simulink model "controlador_multirate"  (R2012b)
settings: Solver=ode3  StartTime=0.0  StopTime=1  FixedStep=1e-5  RelTol=1e-3
model workspace: external: MATLAB File Z:\Work\PLATO\2 - simulador BLDC\3 - Simulador controlador multirate\5 - compacao multirate, sensor MT x sensor M x sensor T\config_simulador_BLDC.m (data not in the file)
undefined symbols (not defined in the file): J, Kd, Ke, Kt, L, Nr, P, R
libraries: simulink x71
(part 1 of 2)
settings Model: Creator=Juliano  LastModifiedBy=Juliano

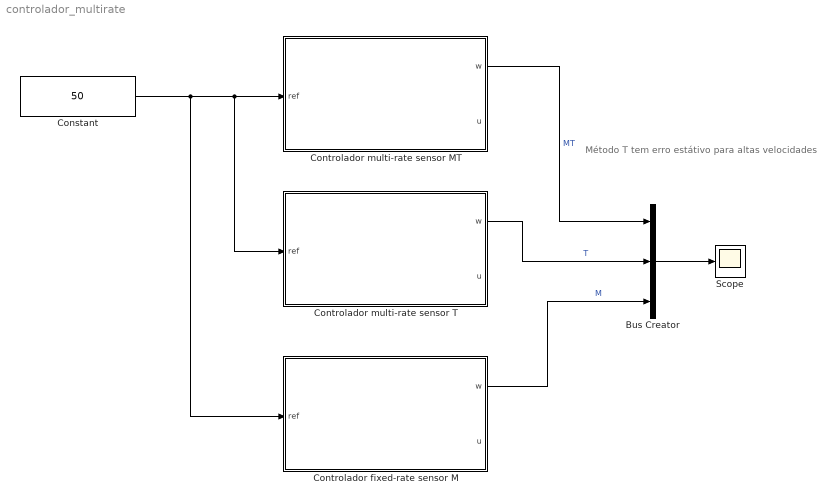
== system controlador_multirate ==
  note: Método T tem erro estátivo para altas velocidades
  Bus Creator : BusCreator  Inputs=3
  Constant : Constant  Value=50
  Controlador fixed-rate sensor M : Subsystem  mask{Ts=0.01}
      mask prompts: Ts "Sample Time"
  Controlador multi-rate sensor MT : Subsystem  mask{Ts=0.01}
      mask prompts: Ts "Sample time inicial do método M/T"
  Controlador multi-rate sensor T : Subsystem  mask{m=10}
      mask prompts: m "Número de pulsos que o método T espera para dar uma estimativa de velocidade (m)"
  Scope : Scope
      settings: TickLabels=on  ShowLegends=on  YMin=5  YMax=85
  wires:
  Constant/1 -> Controlador fixed-rate sensor M/1(ref), Controlador multi-rate sensor T/1(ref), Controlador multi-rate sensor MT/1(ref)
  Controlador multi-rate sensor MT/1(w) -> Bus Creator/1  "MT"
  Controlador fixed-rate sensor M/1(w) -> Bus Creator/3  "M"
  Bus Creator/1 -> Scope/1
  Controlador multi-rate sensor T/1(w) -> Bus Creator/2  "T"

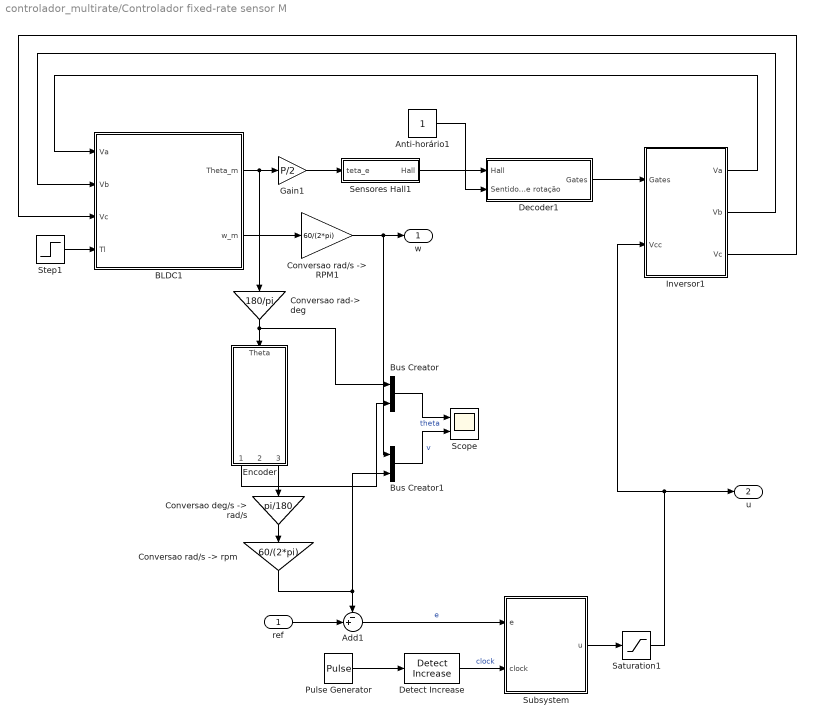
== system controlador_multirate/Controlador fixed-rate sensor M ==
  ref : Inport
  Add1 : Sum  Inputs=-+|
  Anti-horário1 : Constant
  BLDC1 : Subsystem
  Bus Creator : BusCreator  Inputs=2
  Bus Creator1 : BusCreator  Inputs=2
  "Conversao deg/s -> rad/s" : Gain  Gain=pi/180
  Conversao rad-> deg : Gain  Gain=180/pi
  "Conversao rad/s -> RPM1" : Gain  Gain=60/(2*pi)
  "Conversao rad/s -> rpm" : Gain  Gain=60/(2*pi)
  Decoder1 : Subsystem
  Detect Increase : simulink/Logic and Bit Operations/Detect Increase  vinit=0.0  InputProcessing=Inherited  OutDataTypeStr=boolean
  Encoder : Subsystem  mask{Nr=Nr}
      mask prompts: Nr "Número de pulsos por revolução"
  Gain1 : Gain  Gain=P/2
  Inversor1 : Subsystem
  Pulse Generator : DiscretePulseGenerator  PulseType=Time based  Period=Ts  PulseWidth=50
  Saturation1 : Saturate  UpperLimit=12  LowerLimit=-12
  Scope : Scope  NumInputPorts=2
      settings: ShowLegends=on  YMin=0~-350  YMax=400~600
  Sensores Hall1 : Subsystem  AncestorBlock=spsPMSynchronousMachineModel/Discrete Trapezoidal/Hall effect sensor
  Step1 : Step  Time=0.2  After=0*2e-3  SampleTime=0
  Subsystem : Subsystem
  w : Outport
  u : Outport  Port=2
  wires:
  BLDC1/2(w_m) -> "Conversao rad/s -> RPM1"/1
  Inversor1/3(Vc) -> BLDC1/3(Vc)
  Subsystem/1(u) -> Saturation1/1
  Gain1/1 -> Sensores Hall1/1(teta_e)
  "Conversao deg/s -> rad/s"/1 -> "Conversao rad/s -> rpm"/1
  Add1/1 -> Subsystem/1(e)  "e"
  BLDC1/1(Theta_m) -> Gain1/1, Conversao rad-> deg/1
  Step1/1 -> BLDC1/4(Tl)
  Sensores Hall1/1(Hall) -> Decoder1/1("Hall ")
  Inversor1/2(Vb) -> BLDC1/2(Vb)
  Inversor1/1(Va) -> BLDC1/1(Va)
  Decoder1/1(Gates) -> Inversor1/1(Gates)
  Anti-horário1/1 -> Decoder1/2(Sentido de rotação)
  Detect Increase/1 -> Subsystem/2(clock)  "clock"
  Saturation1/1 -> u/1, Inversor1/2(Vcc)
  ref/1 -> Add1/2
  Encoder/3(VelocidadeM) -> "Conversao deg/s -> rad/s"/1
  Pulse Generator/1 -> Detect Increase/1
  Conversao rad-> deg/1 -> Bus Creator/1, Encoder/1(Theta)
  "Conversao rad/s -> rpm"/1 -> Add1/1, Bus Creator1/2
  "Conversao rad/s -> RPM1"/1 -> Bus Creator1/1, w/1
  Encoder/1(Theta_amostrado) -> Bus Creator/2
  Bus Creator/1 -> Scope/1  "theta"
  Bus Creator1/1 -> Scope/2  "v"

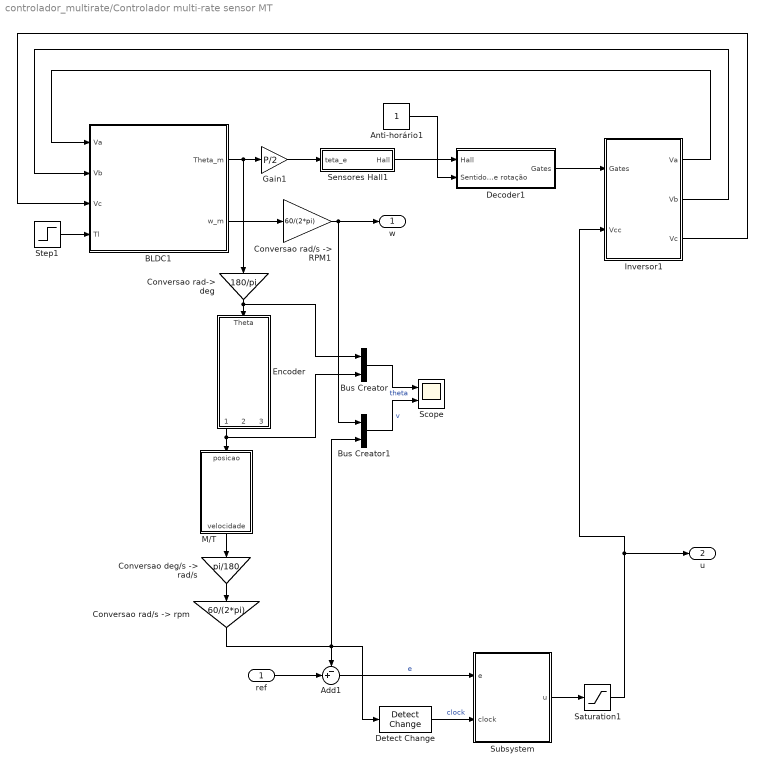
== system controlador_multirate/Controlador multi-rate sensor MT ==
  ref : Inport
  Add1 : Sum  Inputs=-+|
  Anti-horário1 : Constant
  BLDC1 : Subsystem
  Bus Creator : BusCreator  Inputs=2
  Bus Creator1 : BusCreator  Inputs=2
  "Conversao deg/s -> rad/s" : Gain  Gain=pi/180
  Conversao rad-> deg : Gain  Gain=180/pi
  "Conversao rad/s -> RPM1" : Gain  Gain=60/(2*pi)
  "Conversao rad/s -> rpm" : Gain  Gain=60/(2*pi)
  Decoder1 : Subsystem
  Detect Change : simulink/Logic and Bit Operations/Detect Change  vinit=1  InputProcessing=Inherited  OutDataTypeStr=boolean
  Encoder : Subsystem  mask{Nr=Nr}
      mask prompts: Nr "Número de pulsos por revolução"
  Gain1 : Gain  Gain=P/2
  Inversor1 : Subsystem
  M/T : Subsystem  mask{Ts=Ts}
      mask prompts: Ts "Sampling time"
  Saturation1 : Saturate  UpperLimit=12  LowerLimit=-12
  Scope : Scope  NumInputPorts=2
      settings: ShowLegends=on  YMin=0~-350  YMax=400~600  SaveName=ScopeData8
  Sensores Hall1 : Subsystem  AncestorBlock=spsPMSynchronousMachineModel/Discrete Trapezoidal/Hall effect sensor
  Step1 : Step  Time=0.2  After=0*2e-3  SampleTime=0
  Subsystem : Subsystem
  w : Outport
  u : Outport  Port=2
  wires:
  BLDC1/2(w_m) -> "Conversao rad/s -> RPM1"/1
  Inversor1/3(Vc) -> BLDC1/3(Vc)
  Subsystem/1(u) -> Saturation1/1
  Gain1/1 -> Sensores Hall1/1(teta_e)
  "Conversao deg/s -> rad/s"/1 -> "Conversao rad/s -> rpm"/1
  Add1/1 -> Subsystem/1(e)  "e"
  Conversao rad-> deg/1 -> Bus Creator/1, Encoder/1(Theta)
  BLDC1/1(Theta_m) -> Gain1/1, Conversao rad-> deg/1
  Step1/1 -> BLDC1/4(Tl)
  "Conversao rad/s -> rpm"/1 -> Bus Creator1/2, Add1/1, Detect Change/1
  Sensores Hall1/1(Hall) -> Decoder1/1("Hall ")
  Inversor1/2(Vb) -> BLDC1/2(Vb)
  Inversor1/1(Va) -> BLDC1/1(Va)
  Decoder1/1(Gates) -> Inversor1/1(Gates)
  Anti-horário1/1 -> Decoder1/2(Sentido de rotação)
  Detect Change/1 -> Subsystem/2(clock)  "clock"
  Saturation1/1 -> u/1, Inversor1/2(Vcc)
  ref/1 -> Add1/2
  "Conversao rad/s -> RPM1"/1 -> w/1, Bus Creator1/1
  Encoder/1(Theta_amostrado) -> Bus Creator/2, M/T/1(posicao)
  M/T/1(velocidade) -> "Conversao deg/s -> rad/s"/1
  Bus Creator/1 -> Scope/1  "theta"
  Bus Creator1/1 -> Scope/2  "v"

== system controlador_multirate/Controlador multi-rate sensor T ==
  ref : Inport
  Add1 : Sum  Inputs=-+|
  Anti-horário1 : Constant
  BLDC1 : Subsystem
  Bus Creator : BusCreator  Inputs=2
  Bus Creator1 : BusCreator  Inputs=2
  "Conversao deg/s -> rad/s" : Gain  Gain=pi/180
  Conversao rad-> deg : Gain  Gain=180/pi
  "Conversao rad/s -> RPM1" : Gain  Gain=60/(2*pi)
  "Conversao rad/s -> rpm" : Gain  Gain=60/(2*pi)
  Decoder1 : Subsystem
  Detect Change : simulink/Logic and Bit Operations/Detect Change  vinit=1  InputProcessing=Inherited  OutDataTypeStr=boolean
  Encoder : Subsystem  mask{Nr=Nr}
      mask prompts: Nr "Número de pulsos por revolução"
  Gain1 : Gain  Gain=P/2
  Inversor1 : Subsystem
  Saturation1 : Saturate  UpperLimit=12  LowerLimit=-12
  Scope : Scope  NumInputPorts=2
      settings: ShowLegends=on  YMin=0~-400  YMax=275~450  SaveName=ScopeData7
  Sensores Hall1 : Subsystem  AncestorBlock=spsPMSynchronousMachineModel/Discrete Trapezoidal/Hall effect sensor
  Step1 : Step  Time=0.2  After=0*2e-3  SampleTime=0
  Subsystem : Subsystem
  w : Outport
  u : Outport  Port=2
  wires:
  BLDC1/2(w_m) -> "Conversao rad/s -> RPM1"/1
  Inversor1/3(Vc) -> BLDC1/3(Vc)
  Subsystem/1(u) -> Saturation1/1
  Gain1/1 -> Sensores Hall1/1(teta_e)
  "Conversao deg/s -> rad/s"/1 -> "Conversao rad/s -> rpm"/1
  Add1/1 -> Subsystem/1(e)  "e"
  BLDC1/1(Theta_m) -> Gain1/1, Conversao rad-> deg/1
  Step1/1 -> BLDC1/4(Tl)
  "Conversao rad/s -> rpm"/1 -> Bus Creator1/2, Add1/1, Detect Change/1
  Sensores Hall1/1(Hall) -> Decoder1/1("Hall ")
  Inversor1/2(Vb) -> BLDC1/2(Vb)
  Inversor1/1(Va) -> BLDC1/1(Va)
  Decoder1/1(Gates) -> Inversor1/1(Gates)
  Anti-horário1/1 -> Decoder1/2(Sentido de rotação)
  Detect Change/1 -> Subsystem/2(clock)  "clock"
  Saturation1/1 -> u/1, Inversor1/2(Vcc)
  ref/1 -> Add1/2
  Encoder/2(VelocidadeT) -> "Conversao deg/s -> rad/s"/1
  Conversao rad-> deg/1 -> Bus Creator/1, Encoder/1(Theta)
  "Conversao rad/s -> RPM1"/1 -> Bus Creator1/1, w/1
  Encoder/1(Theta_amostrado) -> Bus Creator/2
  Bus Creator/1 -> Scope/1  "theta"
  Bus Creator1/1 -> Scope/2  "v"

== system controlador_multirate/Controlador fixed-rate sensor M/BLDC1 ==
  Va : Inport
  Vb : Inport  Port=2
  Vc : Inport  Port=3
  Tl : Inport  Port=4
  "Cálculo Torque fase \"a\"" : Subsystem
  "Cálculo Torque fase \"b\"" : Subsystem
  "Cálculo Torque fase \"c\"" : Subsystem
  Cálculo das FCEMs : Subsystem
  "Dinâmica fase \"a\"" : Subsystem
  "Dinâmica fase \"b\"" : Subsystem
  "Dinâmica fase \"c\"" : Subsystem
  "Dinâmica mecânica " : Subsystem
  FCEMs : Scope  NumInputPorts=3
      settings: TimeRange=1  YMin=420~-5~-5  YMax=510~5~5  SaveName=ScopeData5
  Gain2 : Gain  Gain=P/2
  Scope : Scope
      settings: TimeRange=1  YMin=420  YMax=510  SaveName=ScopeData4
  Sum : Sum  Inputs=+++
  Vs : Scope  NumInputPorts=3
      settings: TimeRange=1  YMin=420~-5~-5  YMax=510~5~5  SaveName=ScopeData2
  is : Scope  NumInputPorts=3
      settings: TimeRange=1  YMin=420~-5~-5  YMax=510~5~5  SaveName=ScopeData3
  is1 : Scope  NumInputPorts=3
      settings: TimeRange=1  YMin=420~-5~-5  YMax=510~5~5  SaveName=ScopeData6
  Theta_m : Outport
  w_m : Outport  Port=2
  wires:
  Gain2/1 -> "Cálculo Torque fase \"b\""/2(Theta_e), Cálculo das FCEMs/1(Theta_e), "Cálculo Torque fase \"c\""/2(Theta_e), "Cálculo Torque fase \"a\""/2(Theta_e)
  Tl/1 -> "Dinâmica mecânica "/2(Tl)
  "Dinâmica mecânica "/2(w_m) -> w_m/1, Cálculo das FCEMs/2(w_m)  "w_m"
  "Dinâmica mecânica "/1(Theta_m) -> Gain2/1, Theta_m/1  "Theta_m"
  Sum/1 -> "Dinâmica mecânica "/1(Te), Scope/1  "T"
  "Cálculo Torque fase \"c\""/1(T_c) -> Sum/3, is1/3  "T_c"
  "Cálculo Torque fase \"b\""/1(T_b) -> Sum/2, is1/2  "T_b"
  "Cálculo Torque fase \"a\""/1(T_a) -> Sum/1, is1/1  "T_a"
  "Dinâmica fase \"c\""/1(i_c) -> "Cálculo Torque fase \"c\""/1(i_c), is/3  "i_c"
  "Dinâmica fase \"b\""/1(i_b) -> "Cálculo Torque fase \"b\""/1(i_b), is/2  "i_b"
  "Dinâmica fase \"a\""/1(i_a) -> "Cálculo Torque fase \"a\""/1(i_a), is/1  "i_a"
  Vc/1 -> "Dinâmica fase \"c\""/1(Vc), Vs/3
  Vb/1 -> "Dinâmica fase \"b\""/1(Vb), Vs/2
  Va/1 -> "Dinâmica fase \"a\""/1(Va), Vs/1
  Cálculo das FCEMs/3(e_c) -> "Dinâmica fase \"c\""/2(e_c), FCEMs/3  "e_c"
  Cálculo das FCEMs/2(e_b) -> FCEMs/2, "Dinâmica fase \"b\""/2(e_b)  "e_b"
  Cálculo das FCEMs/1(e_a) -> "Dinâmica fase \"a\""/2(e_a), FCEMs/1  "e_a"

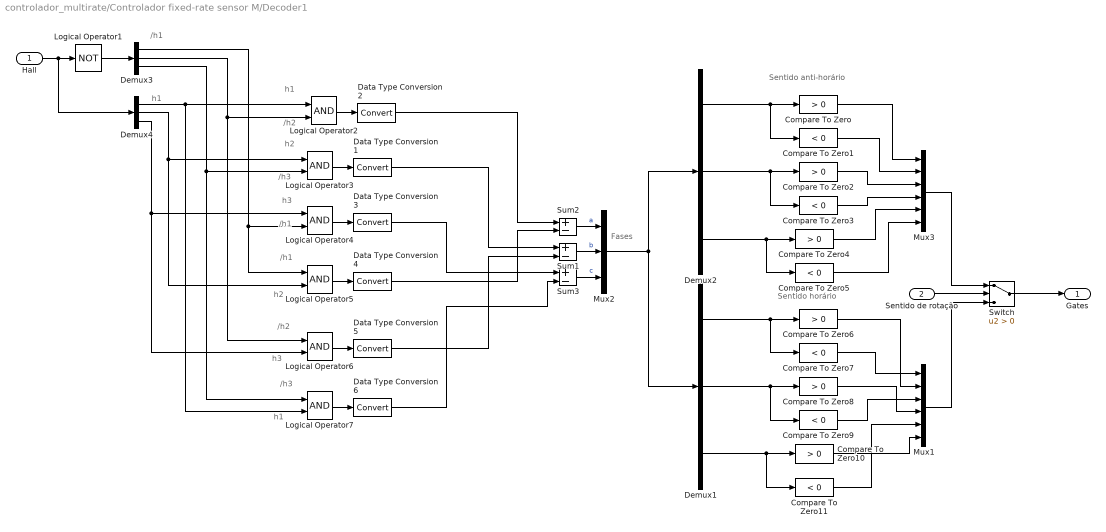
== system controlador_multirate/Controlador fixed-rate sensor M/Decoder1 ==
  note: /h1
  note: h1
  note: h1
  note: /h2
  note: h2
  note: /h3
  note: h3
  note: /h1
  note: /h1
  note: h2
  note: /h2
  note: h3
  note: /h3
  note: h1
  note: Sentido anti-horário
  note: Sentido horário
  note: Fases
  "Hall " : Inport
  Sentido de rotação : Inport  Port=2
  Compare To Zero{,2,4,6,8,10} (6 alike) : simulink/Logic and Bit Operations/Compare To Zero  relop=>  OutDataTypeStr=boolean  ZeroCross=off
  Compare To Zero{1,3,5,7,9,11} (6 alike) : simulink/Logic and Bit Operations/Compare To Zero  relop=<  OutDataTypeStr=boolean  ZeroCross=off
  Data Type Conversion{1..6} (6 alike) : DataTypeConversion
  Demux{1..4} (4 alike) : Demux  Outputs=3
  Logical Operator1 : Logic  Operator=NOT  AllPortsSameDT=off  OutDataTypeStr=boolean
  Logical Operator{2..7} (6 alike) : Logic  AllPortsSameDT=off  OutDataTypeStr=boolean
  Mux1 : Mux  Inputs=6
  Mux2 : Mux  Inputs=3
  Mux3 : Mux  Inputs=6
  Sum1 : Sum  Inputs=+-  OutDataTypeStr=double
  Sum2 : Sum  Inputs=+-  OutDataTypeStr=double
  Sum3 : Sum  Inputs=+-  OutDataTypeStr=double
  Switch : Switch  Criteria=u2 > Threshold
  Gates : Outport
  wires:
  Demux2/1 -> Compare To Zero/1, Compare To Zero1/1
  Demux2/2 -> Compare To Zero2/1, Compare To Zero3/1
  Demux2/3 -> Compare To Zero4/1, Compare To Zero5/1
  Compare To Zero/1 -> Mux3/1
  Compare To Zero1/1 -> Mux3/2
  Compare To Zero2/1 -> Mux3/3
  Compare To Zero3/1 -> Mux3/4
  Compare To Zero4/1 -> Mux3/5
  Compare To Zero5/1 -> Mux3/6
  Demux1/1 -> Compare To Zero6/1, Compare To Zero7/1
  Demux1/2 -> Compare To Zero8/1, Compare To Zero9/1
  Demux1/3 -> Compare To Zero10/1, Compare To Zero11/1
  Mux3/1 -> Switch/1
  Sentido de rotação/1 -> Switch/2
  Mux1/1 -> Switch/3
  Switch/1 -> Gates/1
  Compare To Zero7/1 -> Mux1/1
  Compare To Zero6/1 -> Mux1/2
  Compare To Zero9/1 -> Mux1/3
  Compare To Zero8/1 -> Mux1/4
  Compare To Zero11/1 -> Mux1/5
  Compare To Zero10/1 -> Mux1/6
  "Hall "/1 -> Logical Operator1/1, Demux4/1
  Logical Operator1/1 -> Demux3/1
  Demux4/3 -> Logical Operator4/1, Logical Operator6/2
  Demux4/2 -> Logical Operator3/1, Logical Operator5/2
  Demux4/1 -> Logical Operator2/1, Logical Operator7/2
  Demux3/3 -> Logical Operator3/2, Logical Operator7/1
  Demux3/2 -> Logical Operator2/2, Logical Operator6/1
  Demux3/1 -> Logical Operator4/2, Logical Operator5/1
  Logical Operator2/1 -> Data Type Conversion2/1
  Sum2/1 -> Mux2/1  "a"
  Sum1/1 -> Mux2/2  "b"
  Sum3/1 -> Mux2/3  "c"
  Logical Operator3/1 -> Data Type Conversion1/1
  Logical Operator4/1 -> Data Type Conversion3/1
  Logical Operator5/1 -> Data Type Conversion4/1
  Logical Operator6/1 -> Data Type Conversion5/1
  Logical Operator7/1 -> Data Type Conversion6/1
  Data Type Conversion2/1 -> Sum2/1
  Data Type Conversion4/1 -> Sum2/2
  Data Type Conversion1/1 -> Sum1/1
  Data Type Conversion5/1 -> Sum1/2
  Data Type Conversion3/1 -> Sum3/1
  Data Type Conversion6/1 -> Sum3/2
  Mux2/1 -> Demux2/1, Demux1/1

== system controlador_multirate/Controlador fixed-rate sensor M/Encoder ==
  note: ATENÇÃO: Para o correto funcionamento desse encoder o step size da simulação deve ser menor do que 360/(4*Nr*Vmax),
      | onde Vmax é o valor máximo da derivada do Theta atigindo durante a simulação
  Theta : Inport
  Clock : Clock
  Derivative : Derivative
  Determinar direçao : Subsystem
  Fcn : Fcn  Expr=360/(4*Nr*u)
  Graus / pulso1 : Gain  Gain=360/(4*Nr)  OutDataTypeStr=double
  Memory : Memory  X0=-100
  Método M : Subsystem  mask{Ts=Ts}
      mask prompts: Ts "Sampling time"
  Método T : Subsystem  mask{m=10}
      mask prompts: m "Número de pulsos que o bloco espera para calcular a velocidade média"
  Relational Operator : RelationalOperator  Operator=>  OutDataTypeStr=boolean
  Sensor Óptico : Subsystem
  Sensor Óptico1 : Subsystem
  Stop Simulation : Stop
  Subsystem : Subsystem
  Sum : Sum  Inputs=|+-
  Theta_amostrado : Outport
  VelocidadeT : Outport  Port=2
  VelocidadeM : Outport  Port=3
  wires:
  Método M/1(Velocidade) -> VelocidadeM/1
  Método T/1(Velocidade) -> VelocidadeT/1
  Graus / pulso1/1 -> Theta_amostrado/1, Método T/3(Posição), Método M/1(Posição)
  Subsystem/1(Out) -> Graus / pulso1/1
  Determinar direçao/2(NEG) -> Subsystem/2(NEG)
  Determinar direçao/1(POS) -> Subsystem/1(POS)
  Sensor Óptico1/1(Sinal_Pulso) -> Determinar direçao/2(B), Método T/2(B)  "B"
  Sensor Óptico/1(Sinal_Pulso) -> Método T/1(A), Determinar direçao/1(A)  "A"
  Theta/1 -> Sensor Óptico/1(Theta), Derivative/1, Sensor Óptico1/1(Theta)
  Derivative/1 -> Relational Operator/1
  Clock/1 -> Memory/1, Sum/1
  Memory/1 -> Sum/2
  Sum/1 -> Fcn/1
  Fcn/1 -> Relational Operator/2
  Relational Operator/1 -> Stop Simulation/1

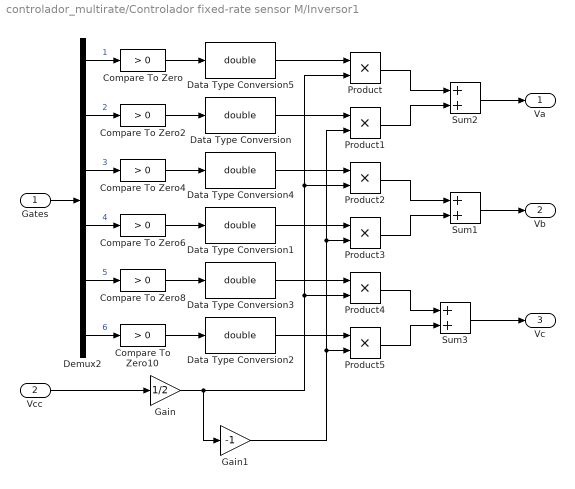
== system controlador_multirate/Controlador fixed-rate sensor M/Inversor1 ==
  Gates : Inport
  Vcc : Inport  Port=2
  Compare To Zero : simulink/Logic and Bit Operations/Compare To Zero  relop=>  OutDataTypeStr=uint8  ZeroCross=off
  Compare To Zero{2,6,8,10} (4 alike) : simulink/Logic and Bit Operations/Compare To Zero  relop=>  OutDataTypeStr=boolean  ZeroCross=off
  Compare To Zero4 : simulink/Logic and Bit Operations/Compare To Zero  relop=>  OutDataTypeStr=uint8  ZeroCross=off
  Data Type Conversion{,1..5} (6 alike) : DataTypeConversion  OutDataTypeStr=double
  Demux2 : Demux  Outputs=6
  Gain : Gain  Gain=1/2
  Gain1 : Gain  Gain=-1
  Product{,1..5} (6 alike) : Product  RndMeth=Zero
  Sum1 : Sum  SaturateOnIntegerOverflow=on
  Sum2 : Sum  SaturateOnIntegerOverflow=on
  Sum3 : Sum  SaturateOnIntegerOverflow=on
  Va : Outport
  Vb : Outport  Port=2
  Vc : Outport  Port=3
  wires:
  Gain/1 -> Product/2, Product2/2, Product4/2, Gain1/1
  Gain1/1 -> Product1/2, Product3/2, Product5/2
  Data Type Conversion5/1 -> Product/1
  Data Type Conversion/1 -> Product1/1
  Data Type Conversion4/1 -> Product2/1
  Data Type Conversion1/1 -> Product3/1
  Data Type Conversion3/1 -> Product4/1
  Data Type Conversion2/1 -> Product5/1
  Product5/1 -> Sum3/2
  Product4/1 -> Sum3/1
  Product3/1 -> Sum1/2
  Product2/1 -> Sum1/1
  Product1/1 -> Sum2/2
  Product/1 -> Sum2/1
  Compare To Zero10/1 -> Data Type Conversion2/1
  Compare To Zero8/1 -> Data Type Conversion3/1
  Compare To Zero6/1 -> Data Type Conversion1/1
  Compare To Zero4/1 -> Data Type Conversion4/1
  Compare To Zero2/1 -> Data Type Conversion/1
  Compare To Zero/1 -> Data Type Conversion5/1
  Demux2/6 -> Compare To Zero10/1  "6"
  Demux2/5 -> Compare To Zero8/1  "5"
  Demux2/4 -> Compare To Zero6/1  "4"
  Demux2/3 -> Compare To Zero4/1  "3"
  Demux2/2 -> Compare To Zero2/1  "2"
  Demux2/1 -> Compare To Zero/1  "1"
  Gates/1 -> Demux2/1
  Sum2/1 -> Va/1
  Sum3/1 -> Vc/1
  Sum1/1 -> Vb/1
  Vcc/1 -> Gain/1

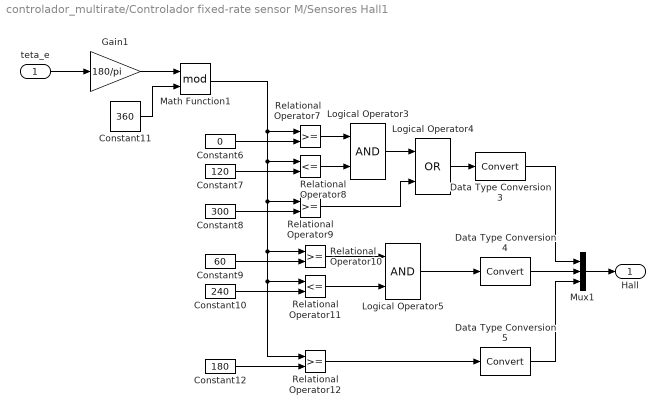
== system controlador_multirate/Controlador fixed-rate sensor M/Sensores Hall1 ==
  teta_e : Inport
  Constant10 : Constant  Value=240
  Constant11 : Constant  Value=360
  Constant12 : Constant  Value=180
  Constant6 : Constant  Value=0
  Constant7 : Constant  Value=120
  Constant8 : Constant  Value=300
  Constant9 : Constant  Value=60
  Data Type Conversion3 : DataTypeConversion  SaturateOnIntegerOverflow=on  RndMeth=Zero
  Data Type Conversion4 : DataTypeConversion  SaturateOnIntegerOverflow=on  RndMeth=Zero
  Data Type Conversion5 : DataTypeConversion  SaturateOnIntegerOverflow=on  RndMeth=Zero
  Gain1 : Gain  Gain=180/pi
  Logical Operator3 : Logic  AllPortsSameDT=off  OutDataTypeStr=boolean
  Logical Operator4 : Logic  Operator=OR  AllPortsSameDT=off  OutDataTypeStr=boolean
  Logical Operator5 : Logic  AllPortsSameDT=off  OutDataTypeStr=boolean
  Math Function1 : Math  Operator=mod  SaturateOnIntegerOverflow=on
  Mux1 : Mux  Inputs=3
  Relational Operator{7,9..10,12} (4 alike) : RelationalOperator  InputSameDT=on
  Relational Operator11 : RelationalOperator  Operator=<=  InputSameDT=on
  Relational Operator8 : RelationalOperator  Operator=<=  InputSameDT=on
  Hall : Outport
  wires:
  Math Function1/1 -> Relational Operator7/1, Relational Operator12/1, Relational Operator11/1, Relational Operator10/1, Relational Operator9/1, Relational Operator8/1
  Constant11/1 -> Math Function1/2
  Gain1/1 -> Math Function1/1
  Relational Operator12/1 -> Data Type Conversion5/1
  Logical Operator5/1 -> Data Type Conversion4/1
  Logical Operator4/1 -> Data Type Conversion3/1
  Data Type Conversion5/1 -> Mux1/3
  Data Type Conversion4/1 -> Mux1/2
  Data Type Conversion3/1 -> Mux1/1
  Mux1/1 -> Hall/1
  Constant12/1 -> Relational Operator12/2
  Constant10/1 -> Relational Operator11/2
  Constant9/1 -> Relational Operator10/2
  Relational Operator11/1 -> Logical Operator5/2
  Relational Operator10/1 -> Logical Operator5/1
  Relational Operator8/1 -> Logical Operator3/2
  Relational Operator7/1 -> Logical Operator3/1
  Logical Operator3/1 -> Logical Operator4/1
  Relational Operator9/1 -> Logical Operator4/2
  Constant8/1 -> Relational Operator9/2
  Constant7/1 -> Relational Operator8/2
  Constant6/1 -> Relational Operator7/2
  teta_e/1 -> Gain1/1

== system controlador_multirate/Controlador fixed-rate sensor M/Subsystem ==
  e : Inport
  clock : Inport  Port=2
  Clock : Clock
  Constant1 : Constant  Value=0.000518155
  Gain2 : Gain  Gain=0.0431726
  Gain3 : Gain  Gain=0.000518155
  Memória controlavel : Subsystem
  Memória controlavel (Y') : Subsystem
  Memória controlavel (e') : Subsystem
  Memória controlavel (u) : Subsystem
  Product : Product  RndMeth=Zero
  Sum : Sum  Inputs=++-
  Sum1 : Sum  Inputs=|+-
  Sum2 : Sum  Inputs=|+-
  u : Outport
  wires:
  e/1 -> Memória controlavel (e')/1(In), Gain3/1
  Memória controlavel (e')/1(Out) -> Product/1
  Memória controlavel (Y')/1(Out) -> Sum/1
  Gain2/1 -> Sum1/2
  clock/1 -> Memória controlavel (u)/2(ctrl), Memória controlavel/2(ctrl), Memória controlavel (e')/2(ctrl), Memória controlavel (Y')/2(ctrl)
  Sum/1 -> Memória controlavel (u)/1(In), Memória controlavel (Y')/1(In)
  Memória controlavel/1(Out) -> Sum2/2
  Product/1 -> Sum/3
  Gain3/1 -> Sum/2
  Clock/1 -> Sum2/1, Memória controlavel/1(In)
  Sum1/1 -> Product/2
  Constant1/1 -> Sum1/1
  Memória controlavel (u)/1(Out) -> u/1
  Sum2/1 -> Gain2/1

== system controlador_multirate/Controlador multi-rate sensor MT/BLDC1 ==
  Va : Inport
  Vb : Inport  Port=2
  Vc : Inport  Port=3
  Tl : Inport  Port=4
  "Cálculo Torque fase \"a\"" : Subsystem
  "Cálculo Torque fase \"b\"" : Subsystem
  "Cálculo Torque fase \"c\"" : Subsystem
  Cálculo das FCEMs : Subsystem
  "Dinâmica fase \"a\"" : Subsystem
  "Dinâmica fase \"b\"" : Subsystem
  "Dinâmica fase \"c\"" : Subsystem
  "Dinâmica mecânica " : Subsystem
  FCEMs : Scope  NumInputPorts=3
      settings: TimeRange=1  YMin=420~-5~-5  YMax=510~5~5  SaveName=ScopeData5
  Gain2 : Gain  Gain=P/2
  Scope : Scope
      settings: TimeRange=1  YMin=420  YMax=510  SaveName=ScopeData4
  Sum : Sum  Inputs=+++
  Vs : Scope  NumInputPorts=3
      settings: TimeRange=1  YMin=420~-5~-5  YMax=510~5~5  SaveName=ScopeData2
  is : Scope  NumInputPorts=3
      settings: TimeRange=1  YMin=420~-5~-5  YMax=510~5~5  SaveName=ScopeData3
  is1 : Scope  NumInputPorts=3
      settings: TimeRange=1  YMin=420~-5~-5  YMax=510~5~5  SaveName=ScopeData6
  Theta_m : Outport
  w_m : Outport  Port=2
  wires:
  Gain2/1 -> "Cálculo Torque fase \"b\""/2(Theta_e), Cálculo das FCEMs/1(Theta_e), "Cálculo Torque fase \"c\""/2(Theta_e), "Cálculo Torque fase \"a\""/2(Theta_e)
  Tl/1 -> "Dinâmica mecânica "/2(Tl)
  "Dinâmica mecânica "/2(w_m) -> w_m/1, Cálculo das FCEMs/2(w_m)  "w_m"
  "Dinâmica mecânica "/1(Theta_m) -> Gain2/1, Theta_m/1  "Theta_m"
  Sum/1 -> "Dinâmica mecânica "/1(Te), Scope/1  "T"
  "Cálculo Torque fase \"c\""/1(T_c) -> Sum/3, is1/3  "T_c"
  "Cálculo Torque fase \"b\""/1(T_b) -> Sum/2, is1/2  "T_b"
  "Cálculo Torque fase \"a\""/1(T_a) -> Sum/1, is1/1  "T_a"
  "Dinâmica fase \"c\""/1(i_c) -> "Cálculo Torque fase \"c\""/1(i_c), is/3  "i_c"
  "Dinâmica fase \"b\""/1(i_b) -> "Cálculo Torque fase \"b\""/1(i_b), is/2  "i_b"
  "Dinâmica fase \"a\""/1(i_a) -> "Cálculo Torque fase \"a\""/1(i_a), is/1  "i_a"
  Vc/1 -> "Dinâmica fase \"c\""/1(Vc), Vs/3
  Vb/1 -> "Dinâmica fase \"b\""/1(Vb), Vs/2
  Va/1 -> "Dinâmica fase \"a\""/1(Va), Vs/1
  Cálculo das FCEMs/3(e_c) -> "Dinâmica fase \"c\""/2(e_c), FCEMs/3  "e_c"
  Cálculo das FCEMs/2(e_b) -> FCEMs/2, "Dinâmica fase \"b\""/2(e_b)  "e_b"
  Cálculo das FCEMs/1(e_a) -> "Dinâmica fase \"a\""/2(e_a), FCEMs/1  "e_a"

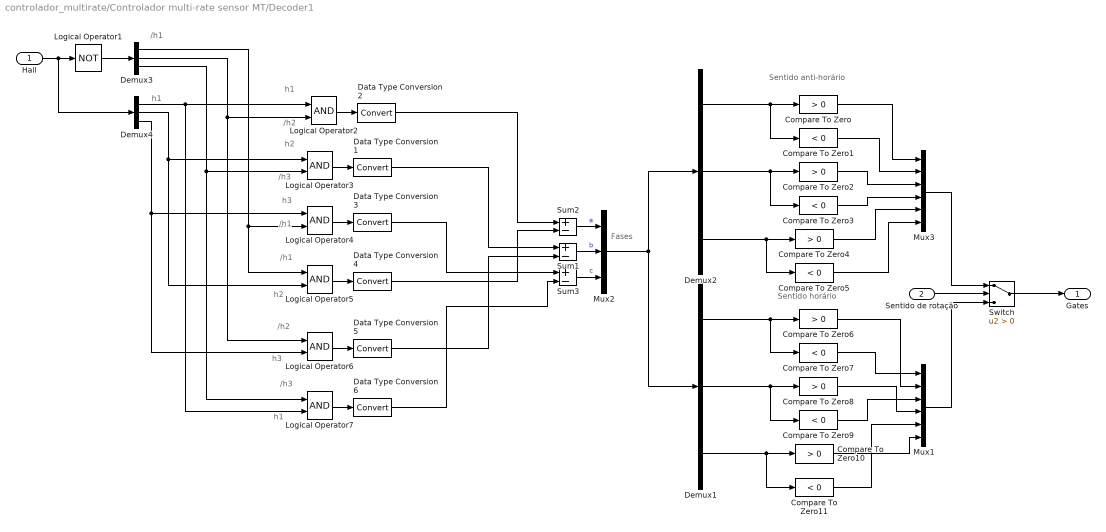
== system controlador_multirate/Controlador multi-rate sensor MT/Decoder1 ==
  note: /h1
  note: h1
  note: h1
  note: /h2
  note: h2
  note: /h3
  note: h3
  note: /h1
  note: /h1
  note: h2
  note: /h2
  note: h3
  note: /h3
  note: h1
  note: Sentido anti-horário
  note: Sentido horário
  note: Fases
  "Hall " : Inport
  Sentido de rotação : Inport  Port=2
  Compare To Zero{,2,4,6,8,10} (6 alike) : simulink/Logic and Bit Operations/Compare To Zero  relop=>  OutDataTypeStr=boolean  ZeroCross=off
  Compare To Zero{1,3,5,7,9,11} (6 alike) : simulink/Logic and Bit Operations/Compare To Zero  relop=<  OutDataTypeStr=boolean  ZeroCross=off
  Data Type Conversion{1..6} (6 alike) : DataTypeConversion
  Demux{1..4} (4 alike) : Demux  Outputs=3
  Logical Operator1 : Logic  Operator=NOT  AllPortsSameDT=off  OutDataTypeStr=boolean
  Logical Operator{2..7} (6 alike) : Logic  AllPortsSameDT=off  OutDataTypeStr=boolean
  Mux1 : Mux  Inputs=6
  Mux2 : Mux  Inputs=3
  Mux3 : Mux  Inputs=6
  Sum1 : Sum  Inputs=+-  OutDataTypeStr=double
  Sum2 : Sum  Inputs=+-  OutDataTypeStr=double
  Sum3 : Sum  Inputs=+-  OutDataTypeStr=double
  Switch : Switch  Criteria=u2 > Threshold
  Gates : Outport
  wires:
  Demux2/1 -> Compare To Zero/1, Compare To Zero1/1
  Demux2/2 -> Compare To Zero2/1, Compare To Zero3/1
  Demux2/3 -> Compare To Zero4/1, Compare To Zero5/1
  Compare To Zero/1 -> Mux3/1
  Compare To Zero1/1 -> Mux3/2
  Compare To Zero2/1 -> Mux3/3
  Compare To Zero3/1 -> Mux3/4
  Compare To Zero4/1 -> Mux3/5
  Compare To Zero5/1 -> Mux3/6
  Demux1/1 -> Compare To Zero6/1, Compare To Zero7/1
  Demux1/2 -> Compare To Zero8/1, Compare To Zero9/1
  Demux1/3 -> Compare To Zero10/1, Compare To Zero11/1
  Mux3/1 -> Switch/1
  Sentido de rotação/1 -> Switch/2
  Mux1/1 -> Switch/3
  Switch/1 -> Gates/1
  Compare To Zero7/1 -> Mux1/1
  Compare To Zero6/1 -> Mux1/2
  Compare To Zero9/1 -> Mux1/3
  Compare To Zero8/1 -> Mux1/4
  Compare To Zero11/1 -> Mux1/5
  Compare To Zero10/1 -> Mux1/6
  "Hall "/1 -> Logical Operator1/1, Demux4/1
  Logical Operator1/1 -> Demux3/1
  Demux4/3 -> Logical Operator4/1, Logical Operator6/2
  Demux4/2 -> Logical Operator3/1, Logical Operator5/2
  Demux4/1 -> Logical Operator2/1, Logical Operator7/2
  Demux3/3 -> Logical Operator3/2, Logical Operator7/1
  Demux3/2 -> Logical Operator2/2, Logical Operator6/1
  Demux3/1 -> Logical Operator4/2, Logical Operator5/1
  Logical Operator2/1 -> Data Type Conversion2/1
  Sum2/1 -> Mux2/1  "a"
  Sum1/1 -> Mux2/2  "b"
  Sum3/1 -> Mux2/3  "c"
  Logical Operator3/1 -> Data Type Conversion1/1
  Logical Operator4/1 -> Data Type Conversion3/1
  Logical Operator5/1 -> Data Type Conversion4/1
  Logical Operator6/1 -> Data Type Conversion5/1
  Logical Operator7/1 -> Data Type Conversion6/1
  Data Type Conversion2/1 -> Sum2/1
  Data Type Conversion4/1 -> Sum2/2
  Data Type Conversion1/1 -> Sum1/1
  Data Type Conversion5/1 -> Sum1/2
  Data Type Conversion3/1 -> Sum3/1
  Data Type Conversion6/1 -> Sum3/2
  Mux2/1 -> Demux2/1, Demux1/1

== system controlador_multirate/Controlador multi-rate sensor MT/Encoder ==
  note: ATENÇÃO: Para o correto funcionamento desse encoder o step size da simulação deve ser menor do que 360/(4*Nr*Vmax),
      | onde Vmax é o valor máximo da derivada do Theta atigindo durante a simulação
  Theta : Inport
  Clock : Clock
  Derivative : Derivative
  Determinar direçao : Subsystem
  Fcn : Fcn  Expr=360/(4*Nr*u)
  Graus / pulso1 : Gain  Gain=360/(4*Nr)  OutDataTypeStr=double
  Memory : Memory  X0=-100
  Método M : Subsystem  mask{Ts=0.1}
      mask prompts: Ts "Sampling time"
  Método T : Subsystem  mask{m=10}
      mask prompts: m "Número de pulsos que o bloco espera para calcular a velocidade média"
  Relational Operator : RelationalOperator  Operator=>  OutDataTypeStr=boolean
  Sensor Óptico : Subsystem
  Sensor Óptico1 : Subsystem
  Stop Simulation : Stop
  Subsystem : Subsystem
  Sum : Sum  Inputs=|+-
  Theta_amostrado : Outport
  VelocidadeT : Outport  Port=2
  VelocidadeM : Outport  Port=3
  wires:
  Método M/1(Velocidade) -> VelocidadeM/1
  Método T/1(Velocidade) -> VelocidadeT/1
  Graus / pulso1/1 -> Theta_amostrado/1, Método T/3(Posição), Método M/1(Posição)
  Subsystem/1(Out) -> Graus / pulso1/1
  Determinar direçao/2(NEG) -> Subsystem/2(NEG)
  Determinar direçao/1(POS) -> Subsystem/1(POS)
  Sensor Óptico1/1(Sinal_Pulso) -> Determinar direçao/2(B), Método T/2(B)  "B"
  Sensor Óptico/1(Sinal_Pulso) -> Método T/1(A), Determinar direçao/1(A)  "A"
  Theta/1 -> Sensor Óptico/1(Theta), Derivative/1, Sensor Óptico1/1(Theta)
  Derivative/1 -> Relational Operator/1
  Clock/1 -> Memory/1, Sum/1
  Memory/1 -> Sum/2
  Sum/1 -> Fcn/1
  Fcn/1 -> Relational Operator/2
  Relational Operator/1 -> Stop Simulation/1

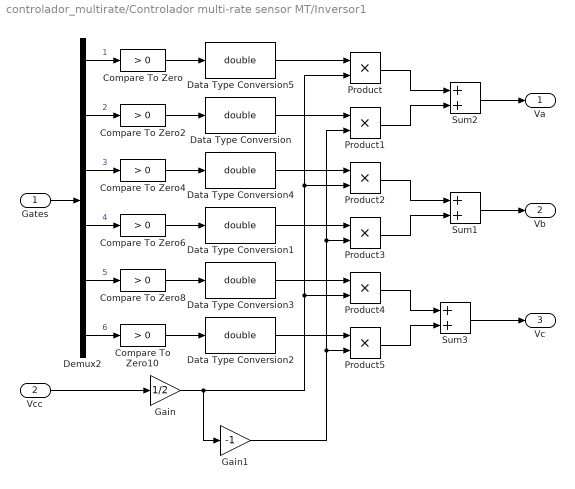
== system controlador_multirate/Controlador multi-rate sensor MT/Inversor1 ==
  Gates : Inport
  Vcc : Inport  Port=2
  Compare To Zero : simulink/Logic and Bit Operations/Compare To Zero  relop=>  OutDataTypeStr=uint8  ZeroCross=off
  Compare To Zero{2,6,8,10} (4 alike) : simulink/Logic and Bit Operations/Compare To Zero  relop=>  OutDataTypeStr=boolean  ZeroCross=off
  Compare To Zero4 : simulink/Logic and Bit Operations/Compare To Zero  relop=>  OutDataTypeStr=uint8  ZeroCross=off
  Data Type Conversion{,1..5} (6 alike) : DataTypeConversion  OutDataTypeStr=double
  Demux2 : Demux  Outputs=6
  Gain : Gain  Gain=1/2
  Gain1 : Gain  Gain=-1
  Product{,1..5} (6 alike) : Product  RndMeth=Zero
  Sum1 : Sum  SaturateOnIntegerOverflow=on
  Sum2 : Sum  SaturateOnIntegerOverflow=on
  Sum3 : Sum  SaturateOnIntegerOverflow=on
  Va : Outport
  Vb : Outport  Port=2
  Vc : Outport  Port=3
  wires:
  Gain/1 -> Product/2, Product2/2, Product4/2, Gain1/1
  Gain1/1 -> Product1/2, Product3/2, Product5/2
  Data Type Conversion5/1 -> Product/1
  Data Type Conversion/1 -> Product1/1
  Data Type Conversion4/1 -> Product2/1
  Data Type Conversion1/1 -> Product3/1
  Data Type Conversion3/1 -> Product4/1
  Data Type Conversion2/1 -> Product5/1
  Product5/1 -> Sum3/2
  Product4/1 -> Sum3/1
  Product3/1 -> Sum1/2
  Product2/1 -> Sum1/1
  Product1/1 -> Sum2/2
  Product/1 -> Sum2/1
  Compare To Zero10/1 -> Data Type Conversion2/1
  Compare To Zero8/1 -> Data Type Conversion3/1
  Compare To Zero6/1 -> Data Type Conversion1/1
  Compare To Zero4/1 -> Data Type Conversion4/1
  Compare To Zero2/1 -> Data Type Conversion/1
  Compare To Zero/1 -> Data Type Conversion5/1
  Demux2/6 -> Compare To Zero10/1  "6"
  Demux2/5 -> Compare To Zero8/1  "5"
  Demux2/4 -> Compare To Zero6/1  "4"
  Demux2/3 -> Compare To Zero4/1  "3"
  Demux2/2 -> Compare To Zero2/1  "2"
  Demux2/1 -> Compare To Zero/1  "1"
  Gates/1 -> Demux2/1
  Sum2/1 -> Va/1
  Sum3/1 -> Vc/1
  Sum1/1 -> Vb/1
  Vcc/1 -> Gain/1

== system controlador_multirate/Controlador multi-rate sensor MT/M//T ==
  posicao : Inport
  Clock : Clock
  Compare To Constant : simulink/Logic and Bit Operations/Compare To Constant  relop=>=  const=Ts  OutDataTypeStr=boolean
  Detect Change : simulink/Logic and Bit Operations/Detect Change  vinit=0  InputProcessing=Inherited  OutDataTypeStr=boolean
  Divide : Product  Inputs=*/
  Logical Operator : Logic  AllPortsSameDT=off  OutDataTypeStr=boolean
  Memória controlavel : Subsystem
  Memória controlavel1 : Subsystem
  Memória controlavel2 : Subsystem
  Sum : Sum  Inputs=+-|
  Sum1 : Sum  Inputs=+-|
  velocidade : Outport
  wires:
  Memória controlavel2/1(Out) -> velocidade/1
  Logical Operator/1 -> Memória controlavel2/2(ctrl), Memória controlavel/2(ctrl), Memória controlavel1/2(ctrl)
  Detect Change/1 -> Logical Operator/1
  Compare To Constant/1 -> Logical Operator/2
  Sum/1 -> Divide/1
  Memória controlavel1/1(Out) -> Sum1/2
  Clock/1 -> Sum1/1, Memória controlavel1/1(In)
  Divide/1 -> Memória controlavel2/1(In)
  Memória controlavel/1(Out) -> Sum/2
  Sum1/1 -> Divide/2, Compare To Constant/1
  posicao/1 -> Memória controlavel/1(In), Sum/1, Detect Change/1

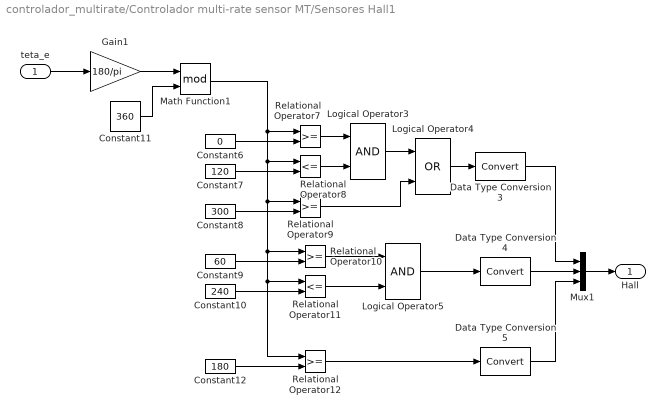
== system controlador_multirate/Controlador multi-rate sensor MT/Sensores Hall1 ==
  teta_e : Inport
  Constant10 : Constant  Value=240
  Constant11 : Constant  Value=360
  Constant12 : Constant  Value=180
  Constant6 : Constant  Value=0
  Constant7 : Constant  Value=120
  Constant8 : Constant  Value=300
  Constant9 : Constant  Value=60
  Data Type Conversion3 : DataTypeConversion  SaturateOnIntegerOverflow=on  RndMeth=Zero
  Data Type Conversion4 : DataTypeConversion  SaturateOnIntegerOverflow=on  RndMeth=Zero
  Data Type Conversion5 : DataTypeConversion  SaturateOnIntegerOverflow=on  RndMeth=Zero
  Gain1 : Gain  Gain=180/pi
  Logical Operator3 : Logic  AllPortsSameDT=off  OutDataTypeStr=boolean
  Logical Operator4 : Logic  Operator=OR  AllPortsSameDT=off  OutDataTypeStr=boolean
  Logical Operator5 : Logic  AllPortsSameDT=off  OutDataTypeStr=boolean
  Math Function1 : Math  Operator=mod  SaturateOnIntegerOverflow=on
  Mux1 : Mux  Inputs=3
  Relational Operator{7,9..10,12} (4 alike) : RelationalOperator  InputSameDT=on
  Relational Operator11 : RelationalOperator  Operator=<=  InputSameDT=on
  Relational Operator8 : RelationalOperator  Operator=<=  InputSameDT=on
  Hall : Outport
  wires:
  Math Function1/1 -> Relational Operator7/1, Relational Operator12/1, Relational Operator11/1, Relational Operator10/1, Relational Operator9/1, Relational Operator8/1
  Constant11/1 -> Math Function1/2
  Gain1/1 -> Math Function1/1
  Relational Operator12/1 -> Data Type Conversion5/1
  Logical Operator5/1 -> Data Type Conversion4/1
  Logical Operator4/1 -> Data Type Conversion3/1
  Data Type Conversion5/1 -> Mux1/3
  Data Type Conversion4/1 -> Mux1/2
  Data Type Conversion3/1 -> Mux1/1
  Mux1/1 -> Hall/1
  Constant12/1 -> Relational Operator12/2
  Constant10/1 -> Relational Operator11/2
  Constant9/1 -> Relational Operator10/2
  Relational Operator11/1 -> Logical Operator5/2
  Relational Operator10/1 -> Logical Operator5/1
  Relational Operator8/1 -> Logical Operator3/2
  Relational Operator7/1 -> Logical Operator3/1
  Logical Operator3/1 -> Logical Operator4/1
  Relational Operator9/1 -> Logical Operator4/2
  Constant8/1 -> Relational Operator9/2
  Constant7/1 -> Relational Operator8/2
  Constant6/1 -> Relational Operator7/2
  teta_e/1 -> Gain1/1

== system controlador_multirate/Controlador multi-rate sensor MT/Subsystem ==
  e : Inport
  clock : Inport  Port=2
  Clock : Clock
  Constant1 : Constant  Value=0.000518155
  Gain2 : Gain  Gain=0.0431726
  Gain3 : Gain  Gain=0.000518155
  Memória controlavel : Subsystem
  Memória controlavel (Y') : Subsystem
  Memória controlavel (e') : Subsystem
  Memória controlavel (u) : Subsystem
  Product : Product  RndMeth=Zero
  Sum : Sum  Inputs=++-
  Sum1 : Sum  Inputs=|+-
  Sum2 : Sum  Inputs=|+-
  u : Outport
  wires:
  e/1 -> Memória controlavel (e')/1(In), Gain3/1
  Memória controlavel (e')/1(Out) -> Product/1
  Memória controlavel (Y')/1(Out) -> Sum/1
  Gain2/1 -> Sum1/2
  clock/1 -> Memória controlavel (u)/2(ctrl), Memória controlavel/2(ctrl), Memória controlavel (e')/2(ctrl), Memória controlavel (Y')/2(ctrl)
  Sum/1 -> Memória controlavel (u)/1(In), Memória controlavel (Y')/1(In)
  Memória controlavel/1(Out) -> Sum2/2
  Product/1 -> Sum/3
  Gain3/1 -> Sum/2
  Clock/1 -> Sum2/1, Memória controlavel/1(In)
  Sum1/1 -> Product/2
  Constant1/1 -> Sum1/1
  Memória controlavel (u)/1(Out) -> u/1
  Sum2/1 -> Gain2/1

== system controlador_multirate/Controlador multi-rate sensor T/BLDC1 ==
  Va : Inport
  Vb : Inport  Port=2
  Vc : Inport  Port=3
  Tl : Inport  Port=4
  "Cálculo Torque fase \"a\"" : Subsystem
  "Cálculo Torque fase \"b\"" : Subsystem
  "Cálculo Torque fase \"c\"" : Subsystem
  Cálculo das FCEMs : Subsystem
  "Dinâmica fase \"a\"" : Subsystem
  "Dinâmica fase \"b\"" : Subsystem
  "Dinâmica fase \"c\"" : Subsystem
  "Dinâmica mecânica " : Subsystem
  FCEMs : Scope  NumInputPorts=3
      settings: TimeRange=1  YMin=420~-5~-5  YMax=510~5~5  SaveName=ScopeData5
  Gain2 : Gain  Gain=P/2
  Scope : Scope
      settings: TimeRange=1  YMin=420  YMax=510  SaveName=ScopeData4
  Sum : Sum  Inputs=+++
  Vs : Scope  NumInputPorts=3
      settings: TimeRange=1  YMin=420~-5~-5  YMax=510~5~5  SaveName=ScopeData2
  is : Scope  NumInputPorts=3
      settings: TimeRange=1  YMin=420~-5~-5  YMax=510~5~5  SaveName=ScopeData3
  is1 : Scope  NumInputPorts=3
      settings: TimeRange=1  YMin=420~-5~-5  YMax=510~5~5  SaveName=ScopeData6
  Theta_m : Outport
  w_m : Outport  Port=2
  wires:
  Gain2/1 -> "Cálculo Torque fase \"b\""/2(Theta_e), Cálculo das FCEMs/1(Theta_e), "Cálculo Torque fase \"c\""/2(Theta_e), "Cálculo Torque fase \"a\""/2(Theta_e)
  Tl/1 -> "Dinâmica mecânica "/2(Tl)
  "Dinâmica mecânica "/2(w_m) -> w_m/1, Cálculo das FCEMs/2(w_m)  "w_m"
  "Dinâmica mecânica "/1(Theta_m) -> Gain2/1, Theta_m/1  "Theta_m"
  Sum/1 -> "Dinâmica mecânica "/1(Te), Scope/1  "T"
  "Cálculo Torque fase \"c\""/1(T_c) -> Sum/3, is1/3  "T_c"
  "Cálculo Torque fase \"b\""/1(T_b) -> Sum/2, is1/2  "T_b"
  "Cálculo Torque fase \"a\""/1(T_a) -> Sum/1, is1/1  "T_a"
  "Dinâmica fase \"c\""/1(i_c) -> "Cálculo Torque fase \"c\""/1(i_c), is/3  "i_c"
  "Dinâmica fase \"b\""/1(i_b) -> "Cálculo Torque fase \"b\""/1(i_b), is/2  "i_b"
  "Dinâmica fase \"a\""/1(i_a) -> "Cálculo Torque fase \"a\""/1(i_a), is/1  "i_a"
  Vc/1 -> "Dinâmica fase \"c\""/1(Vc), Vs/3
  Vb/1 -> "Dinâmica fase \"b\""/1(Vb), Vs/2
  Va/1 -> "Dinâmica fase \"a\""/1(Va), Vs/1
  Cálculo das FCEMs/3(e_c) -> "Dinâmica fase \"c\""/2(e_c), FCEMs/3  "e_c"
  Cálculo das FCEMs/2(e_b) -> FCEMs/2, "Dinâmica fase \"b\""/2(e_b)  "e_b"
  Cálculo das FCEMs/1(e_a) -> "Dinâmica fase \"a\""/2(e_a), FCEMs/1  "e_a"

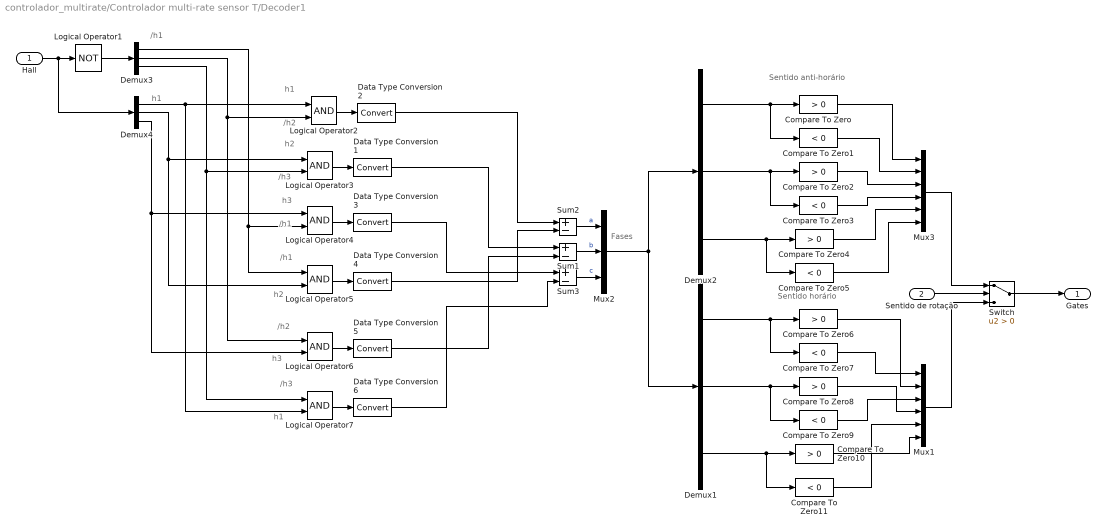
== system controlador_multirate/Controlador multi-rate sensor T/Decoder1 ==
  note: /h1
  note: h1
  note: h1
  note: /h2
  note: h2
  note: /h3
  note: h3
  note: /h1
  note: /h1
  note: h2
  note: /h2
  note: h3
  note: /h3
  note: h1
  note: Sentido anti-horário
  note: Sentido horário
  note: Fases
  "Hall " : Inport
  Sentido de rotação : Inport  Port=2
  Compare To Zero{,2,4,6,8,10} (6 alike) : simulink/Logic and Bit Operations/Compare To Zero  relop=>  OutDataTypeStr=boolean  ZeroCross=off
  Compare To Zero{1,3,5,7,9,11} (6 alike) : simulink/Logic and Bit Operations/Compare To Zero  relop=<  OutDataTypeStr=boolean  ZeroCross=off
  Data Type Conversion{1..6} (6 alike) : DataTypeConversion
  Demux{1..4} (4 alike) : Demux  Outputs=3
  Logical Operator1 : Logic  Operator=NOT  AllPortsSameDT=off  OutDataTypeStr=boolean
  Logical Operator{2..7} (6 alike) : Logic  AllPortsSameDT=off  OutDataTypeStr=boolean
  Mux1 : Mux  Inputs=6
  Mux2 : Mux  Inputs=3
  Mux3 : Mux  Inputs=6
  Sum1 : Sum  Inputs=+-  OutDataTypeStr=double
  Sum2 : Sum  Inputs=+-  OutDataTypeStr=double
  Sum3 : Sum  Inputs=+-  OutDataTypeStr=double
  Switch : Switch  Criteria=u2 > Threshold
  Gates : Outport
  wires:
  Demux2/1 -> Compare To Zero/1, Compare To Zero1/1
  Demux2/2 -> Compare To Zero2/1, Compare To Zero3/1
  Demux2/3 -> Compare To Zero4/1, Compare To Zero5/1
  Compare To Zero/1 -> Mux3/1
  Compare To Zero1/1 -> Mux3/2
  Compare To Zero2/1 -> Mux3/3
  Compare To Zero3/1 -> Mux3/4
  Compare To Zero4/1 -> Mux3/5
  Compare To Zero5/1 -> Mux3/6
  Demux1/1 -> Compare To Zero6/1, Compare To Zero7/1
  Demux1/2 -> Compare To Zero8/1, Compare To Zero9/1
  Demux1/3 -> Compare To Zero10/1, Compare To Zero11/1
  Mux3/1 -> Switch/1
  Sentido de rotação/1 -> Switch/2
  Mux1/1 -> Switch/3
  Switch/1 -> Gates/1
  Compare To Zero7/1 -> Mux1/1
  Compare To Zero6/1 -> Mux1/2
  Compare To Zero9/1 -> Mux1/3
  Compare To Zero8/1 -> Mux1/4
  Compare To Zero11/1 -> Mux1/5
  Compare To Zero10/1 -> Mux1/6
  "Hall "/1 -> Logical Operator1/1, Demux4/1
  Logical Operator1/1 -> Demux3/1
  Demux4/3 -> Logical Operator4/1, Logical Operator6/2
  Demux4/2 -> Logical Operator3/1, Logical Operator5/2
  Demux4/1 -> Logical Operator2/1, Logical Operator7/2
  Demux3/3 -> Logical Operator3/2, Logical Operator7/1
  Demux3/2 -> Logical Operator2/2, Logical Operator6/1
  Demux3/1 -> Logical Operator4/2, Logical Operator5/1
  Logical Operator2/1 -> Data Type Conversion2/1
  Sum2/1 -> Mux2/1  "a"
  Sum1/1 -> Mux2/2  "b"
  Sum3/1 -> Mux2/3  "c"
  Logical Operator3/1 -> Data Type Conversion1/1
  Logical Operator4/1 -> Data Type Conversion3/1
  Logical Operator5/1 -> Data Type Conversion4/1
  Logical Operator6/1 -> Data Type Conversion5/1
  Logical Operator7/1 -> Data Type Conversion6/1
  Data Type Conversion2/1 -> Sum2/1
  Data Type Conversion4/1 -> Sum2/2
  Data Type Conversion1/1 -> Sum1/1
  Data Type Conversion5/1 -> Sum1/2
  Data Type Conversion3/1 -> Sum3/1
  Data Type Conversion6/1 -> Sum3/2
  Mux2/1 -> Demux2/1, Demux1/1

== system controlador_multirate/Controlador multi-rate sensor T/Encoder ==
  note: ATENÇÃO: Para o correto funcionamento desse encoder o step size da simulação deve ser menor do que 360/(4*Nr*Vmax),
      | onde Vmax é o valor máximo da derivada do Theta atigindo durante a simulação
  Theta : Inport
  Clock : Clock
  Derivative : Derivative
  Determinar direçao : Subsystem
  Fcn : Fcn  Expr=360/(4*Nr*u)
  Graus / pulso1 : Gain  Gain=360/(4*Nr)  OutDataTypeStr=double
  Memory : Memory  X0=-100
  Método M : Subsystem  mask{Ts=0.1}
      mask prompts: Ts "Sampling time"
  Método T : Subsystem  mask{m=m}
      mask prompts: m "Número de pulsos que o bloco espera para calcular a velocidade média"
  Relational Operator : RelationalOperator  Operator=>  OutDataTypeStr=boolean
  Sensor Óptico : Subsystem
  Sensor Óptico1 : Subsystem
  Stop Simulation : Stop
  Subsystem : Subsystem
  Sum : Sum  Inputs=|+-
  Theta_amostrado : Outport
  VelocidadeT : Outport  Port=2
  VelocidadeM : Outport  Port=3
  wires:
  Método M/1(Velocidade) -> VelocidadeM/1
  Método T/1(Velocidade) -> VelocidadeT/1
  Graus / pulso1/1 -> Theta_amostrado/1, Método T/3(Posição), Método M/1(Posição)
  Subsystem/1(Out) -> Graus / pulso1/1
  Determinar direçao/2(NEG) -> Subsystem/2(NEG)
  Determinar direçao/1(POS) -> Subsystem/1(POS)
  Sensor Óptico1/1(Sinal_Pulso) -> Determinar direçao/2(B), Método T/2(B)  "B"
  Sensor Óptico/1(Sinal_Pulso) -> Método T/1(A), Determinar direçao/1(A)  "A"
  Theta/1 -> Sensor Óptico/1(Theta), Sensor Óptico1/1(Theta), Derivative/1
  Derivative/1 -> Relational Operator/1
  Clock/1 -> Memory/1, Sum/1
  Memory/1 -> Sum/2
  Sum/1 -> Fcn/1
  Fcn/1 -> Relational Operator/2
  Relational Operator/1 -> Stop Simulation/1

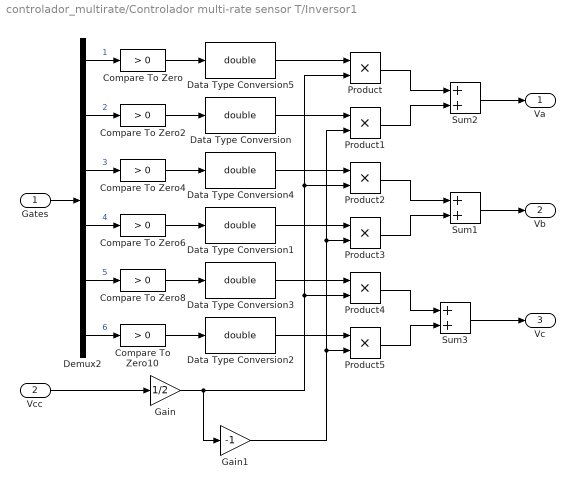
== system controlador_multirate/Controlador multi-rate sensor T/Inversor1 ==
  Gates : Inport
  Vcc : Inport  Port=2
  Compare To Zero : simulink/Logic and Bit Operations/Compare To Zero  relop=>  OutDataTypeStr=uint8  ZeroCross=off
  Compare To Zero{2,6,8,10} (4 alike) : simulink/Logic and Bit Operations/Compare To Zero  relop=>  OutDataTypeStr=boolean  ZeroCross=off
  Compare To Zero4 : simulink/Logic and Bit Operations/Compare To Zero  relop=>  OutDataTypeStr=uint8  ZeroCross=off
  Data Type Conversion{,1..5} (6 alike) : DataTypeConversion  OutDataTypeStr=double
  Demux2 : Demux  Outputs=6
  Gain : Gain  Gain=1/2
  Gain1 : Gain  Gain=-1
  Product{,1..5} (6 alike) : Product  RndMeth=Zero
  Sum1 : Sum  SaturateOnIntegerOverflow=on
  Sum2 : Sum  SaturateOnIntegerOverflow=on
  Sum3 : Sum  SaturateOnIntegerOverflow=on
  Va : Outport
  Vb : Outport  Port=2
  Vc : Outport  Port=3
  wires:
  Gain/1 -> Product/2, Product2/2, Product4/2, Gain1/1
  Gain1/1 -> Product1/2, Product3/2, Product5/2
  Data Type Conversion5/1 -> Product/1
  Data Type Conversion/1 -> Product1/1
  Data Type Conversion4/1 -> Product2/1
  Data Type Conversion1/1 -> Product3/1
  Data Type Conversion3/1 -> Product4/1
  Data Type Conversion2/1 -> Product5/1
  Product5/1 -> Sum3/2
  Product4/1 -> Sum3/1
  Product3/1 -> Sum1/2
  Product2/1 -> Sum1/1
  Product1/1 -> Sum2/2
  Product/1 -> Sum2/1
  Compare To Zero10/1 -> Data Type Conversion2/1
  Compare To Zero8/1 -> Data Type Conversion3/1
  Compare To Zero6/1 -> Data Type Conversion1/1
  Compare To Zero4/1 -> Data Type Conversion4/1
  Compare To Zero2/1 -> Data Type Conversion/1
  Compare To Zero/1 -> Data Type Conversion5/1
  Demux2/6 -> Compare To Zero10/1  "6"
  Demux2/5 -> Compare To Zero8/1  "5"
  Demux2/4 -> Compare To Zero6/1  "4"
  Demux2/3 -> Compare To Zero4/1  "3"
  Demux2/2 -> Compare To Zero2/1  "2"
  Demux2/1 -> Compare To Zero/1  "1"
  Gates/1 -> Demux2/1
  Sum2/1 -> Va/1
  Sum3/1 -> Vc/1
  Sum1/1 -> Vb/1
  Vcc/1 -> Gain/1

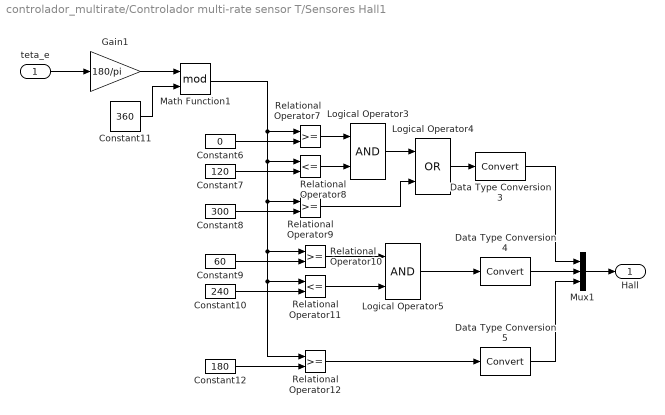
== system controlador_multirate/Controlador multi-rate sensor T/Sensores Hall1 ==
  teta_e : Inport
  Constant10 : Constant  Value=240
  Constant11 : Constant  Value=360
  Constant12 : Constant  Value=180
  Constant6 : Constant  Value=0
  Constant7 : Constant  Value=120
  Constant8 : Constant  Value=300
  Constant9 : Constant  Value=60
  Data Type Conversion3 : DataTypeConversion  SaturateOnIntegerOverflow=on  RndMeth=Zero
  Data Type Conversion4 : DataTypeConversion  SaturateOnIntegerOverflow=on  RndMeth=Zero
  Data Type Conversion5 : DataTypeConversion  SaturateOnIntegerOverflow=on  RndMeth=Zero
  Gain1 : Gain  Gain=180/pi
  Logical Operator3 : Logic  AllPortsSameDT=off  OutDataTypeStr=boolean
  Logical Operator4 : Logic  Operator=OR  AllPortsSameDT=off  OutDataTypeStr=boolean
  Logical Operator5 : Logic  AllPortsSameDT=off  OutDataTypeStr=boolean
  Math Function1 : Math  Operator=mod  SaturateOnIntegerOverflow=on
  Mux1 : Mux  Inputs=3
  Relational Operator{7,9..10,12} (4 alike) : RelationalOperator  InputSameDT=on
  Relational Operator11 : RelationalOperator  Operator=<=  InputSameDT=on
  Relational Operator8 : RelationalOperator  Operator=<=  InputSameDT=on
  Hall : Outport
  wires:
  Math Function1/1 -> Relational Operator7/1, Relational Operator12/1, Relational Operator11/1, Relational Operator10/1, Relational Operator9/1, Relational Operator8/1
  Constant11/1 -> Math Function1/2
  Gain1/1 -> Math Function1/1
  Relational Operator12/1 -> Data Type Conversion5/1
  Logical Operator5/1 -> Data Type Conversion4/1
  Logical Operator4/1 -> Data Type Conversion3/1
  Data Type Conversion5/1 -> Mux1/3
  Data Type Conversion4/1 -> Mux1/2
  Data Type Conversion3/1 -> Mux1/1
  Mux1/1 -> Hall/1
  Constant12/1 -> Relational Operator12/2
  Constant10/1 -> Relational Operator11/2
  Constant9/1 -> Relational Operator10/2
  Relational Operator11/1 -> Logical Operator5/2
  Relational Operator10/1 -> Logical Operator5/1
  Relational Operator8/1 -> Logical Operator3/2
  Relational Operator7/1 -> Logical Operator3/1
  Logical Operator3/1 -> Logical Operator4/1
  Relational Operator9/1 -> Logical Operator4/2
  Constant8/1 -> Relational Operator9/2
  Constant7/1 -> Relational Operator8/2
  Constant6/1 -> Relational Operator7/2
  teta_e/1 -> Gain1/1

== system controlador_multirate/Controlador multi-rate sensor T/Subsystem ==
  e : Inport
  clock : Inport  Port=2
  Clock : Clock
  Constant1 : Constant  Value=0.000518155
  Gain2 : Gain  Gain=0.0431726
  Gain3 : Gain  Gain=0.000518155
  Memória controlavel : Subsystem
  Memória controlavel (Y') : Subsystem
  Memória controlavel (e') : Subsystem
  Memória controlavel (u) : Subsystem
  Product : Product  RndMeth=Zero
  Sum : Sum  Inputs=++-
  Sum1 : Sum  Inputs=|+-
  Sum2 : Sum  Inputs=|+-
  u : Outport
  wires:
  e/1 -> Memória controlavel (e')/1(In), Gain3/1
  Memória controlavel (e')/1(Out) -> Product/1
  Memória controlavel (Y')/1(Out) -> Sum/1
  Gain2/1 -> Sum1/2
  clock/1 -> Memória controlavel (u)/2(ctrl), Memória controlavel/2(ctrl), Memória controlavel (e')/2(ctrl), Memória controlavel (Y')/2(ctrl)
  Sum/1 -> Memória controlavel (u)/1(In), Memória controlavel (Y')/1(In)
  Memória controlavel/1(Out) -> Sum2/2
  Product/1 -> Sum/3
  Gain3/1 -> Sum/2
  Clock/1 -> Sum2/1, Memória controlavel/1(In)
  Sum1/1 -> Product/2
  Constant1/1 -> Sum1/1
  Memória controlavel (u)/1(Out) -> u/1
  Sum2/1 -> Gain2/1

== system controlador_multirate/Controlador fixed-rate sensor M/BLDC1/Cálculo Torque fase "a" ==
  i_a : Inport
  Theta_e : Inport  Port=2
  Constant1 : Constant  Value=360
  Gain : Gain  Gain=Kt/2
  Gain1 : Gain  Gain=180/pi
  Math Function1 : Math  Operator=mod  SaturateOnIntegerOverflow=on
  Product : Product  RndMeth=Zero
  fa1 : Lookup  InputValues=[0 30 60 90 120 150 180 210 240 270 300 330 360]  Table=[ 1 1 1 0 -1 -1 -1 -1 -1 0 1 1 1]
  T_a : Outport
  wires:
  Constant1/1 -> Math Function1/2
  Gain1/1 -> Math Function1/1
  Product/1 -> T_a/1
  fa1/1 -> Product/1
  Theta_e/1 -> Gain1/1
  Math Function1/1 -> fa1/1
  Gain/1 -> Product/2
  i_a/1 -> Gain/1

== system controlador_multirate/Controlador fixed-rate sensor M/BLDC1/Cálculo Torque fase "b" ==
  i_b : Inport
  Theta_e : Inport  Port=2
  Constant1 : Constant  Value=360
  Gain : Gain  Gain=Kt/2
  Gain1 : Gain  Gain=180/pi
  Math Function1 : Math  Operator=mod  SaturateOnIntegerOverflow=on
  Product : Product  RndMeth=Zero
  fb2 : Lookup  InputValues=[0 30 60 90 120 150 180 210 240 270 300 330 360]  Table=[-1 0 1 1 1 1 1 0 -1 -1 -1 -1 -1]
  T_b : Outport
  wires:
  Constant1/1 -> Math Function1/2
  Gain1/1 -> Math Function1/1
  i_b/1 -> Gain/1
  Gain/1 -> Product/2
  Math Function1/1 -> fb2/1
  Theta_e/1 -> Gain1/1
  fb2/1 -> Product/1
  Product/1 -> T_b/1

== system controlador_multirate/Controlador fixed-rate sensor M/BLDC1/Cálculo Torque fase "c" ==
  i_c : Inport
  Theta_e : Inport  Port=2
  Constant1 : Constant  Value=360
  Gain : Gain  Gain=Kt/2
  Gain1 : Gain  Gain=180/pi
  Math Function1 : Math  Operator=mod  SaturateOnIntegerOverflow=on
  Product : Product  RndMeth=Zero
  fc1 : Lookup  InputValues=[0 30 60 90 120 150 180 210 240 270 300 330 360]  Table=[-1 -1 -1 -1 -1 0 1 1 1 1 1 0 -1]
  T_c : Outport
  wires:
  Constant1/1 -> Math Function1/2
  Gain1/1 -> Math Function1/1
  Product/1 -> T_c/1
  fc1/1 -> Product/1
  Theta_e/1 -> Gain1/1
  Math Function1/1 -> fc1/1
  Gain/1 -> Product/2
  i_c/1 -> Gain/1

== system controlador_multirate/Controlador fixed-rate sensor M/BLDC1/Cálculo das FCEMs ==
  Theta_e : Inport
  w_m : Inport  Port=2
  Constant1 : Constant  Value=360
  Constant2 : Constant  Value=360
  Constant3 : Constant  Value=360
  Gain1 : Gain  Gain=180/pi
  Gain2 : Gain  Gain=Ke/2
  Gain3 : Gain  Gain=Ke/2
  Gain4 : Gain  Gain=Ke/2
  Gain5 : Gain  Gain=180/pi
  Gain6 : Gain  Gain=180/pi
  Math Function1 : Math  Operator=mod  SaturateOnIntegerOverflow=on
  Math Function2 : Math  Operator=mod  SaturateOnIntegerOverflow=on
  Math Function3 : Math  Operator=mod  SaturateOnIntegerOverflow=on
  Product : Product  RndMeth=Zero
  Product1 : Product  RndMeth=Zero
  Product2 : Product  RndMeth=Zero
  fa1 : Lookup  InputValues=[0 30 60 90 120 150 180 210 240 270 300 330 360]  Table=[ 1 1 1 0 -1 -1 -1 -1 -1 0 1 1 1]
  fb2 : Lookup  InputValues=[0 30 60 90 120 150 180 210 240 270 300 330 360]  Table=[-1 0 1 1 1 1 1 0 -1 -1 -1 -1 -1]
  fc1 : Lookup  InputValues=[0 30 60 90 120 150 180 210 240 270 300 330 360]  Table=[-1 -1 -1 -1 -1 0 1 1 1 1 1 0 -1]
  e_a : Outport
  e_b : Outport  Port=2
  e_c : Outport  Port=3
  wires:
  Constant3/1 -> Math Function3/2
  Constant2/1 -> Math Function2/2
  Constant1/1 -> Math Function1/2
  Product/1 -> e_a/1
  Product1/1 -> e_b/1
  Theta_e/1 -> Gain5/1, Gain1/1, Gain6/1
  Product2/1 -> e_c/1
  Gain2/1 -> Product/2
  w_m/1 -> Product/1, Product1/1, Product2/1
  Gain3/1 -> Product1/2
  Gain4/1 -> Product2/2
  Gain1/1 -> Math Function1/1
  Gain5/1 -> Math Function2/1
  Gain6/1 -> Math Function3/1
  Math Function1/1 -> fa1/1
  fa1/1 -> Gain2/1
  Math Function2/1 -> fb2/1
  fb2/1 -> Gain3/1
  Math Function3/1 -> fc1/1
  fc1/1 -> Gain4/1
